simulink model "simulation_ex_4_2014a"  (R2014a)
settings: Solver=ode45  SolverMode=SingleTasking  StartTime=0.0  StopTime=3000  RelTol=1e-3
settings Model: CovMetricSettings=dwe  CovHtmlReporting=off  covSaveCumulativeToWorkspaceVar=off  CovSaveSingleToWorkspaceVar=off  CovExternalEMLEnable=on  CovSFcnEnable=on  Creator=HanO  LastModifiedBy=HanO
settings DataIOCC: LimitDataPoints=off  SaveFormat=StructureWithTime  ReturnWorkspaceOutputs=on
settings DebuggingCC: MergeDetectMultiDrivingBlocksExec=error  SolverPrmCheckMsg=none  FrameProcessingCompatibilityMsg=error  SFUnexpectedBacktrackingDiag=error  SFNoUnconditionalDefaultTransitionDiag=error
settings HardwareCC: ProdBitPerPointer=64  ProdLargestAtomicFloat=Float  ProdIntDivRoundTo=Zero  ProdEndianess=LittleEndian  ProdHWDeviceType=Specified
settings ModelReferenceCC: PropagateSignalLabelsOutOfModel=on
settings SFSimCC: SimUseLocalCustomCode=on
settings RTWCC: RTWUseLocalCustomCode=on
settings GRTTargetCC: TargetLangStandard=C99 (ISO)

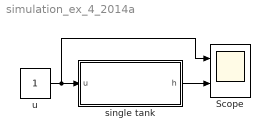
== system simulation_ex_4_2014a ==
  Scope : Scope  NumInputPorts=2
      settings: TimeRange=auto  MaxDataPoints=5000  SaveName=ScopeData  YMin=0.9~-0.19266  YMax=1.1~2.24363  SampleTime=-1
  single tank : Subsystem  mask{AA=50, a=0.5, k=0.1, Cd=0.2, g=9.81, h0=2}
      mask prompts: AA "Tiết diện ngang bồn chứa A ="; a "Tiết diện van xả a ="; k "Hệ số tỉ lệ công suất máy bơm k ="; Cd "Hệ số xả Cd ="; g "Gia tốc trọng trường g ="; h0 "Mực nước ban đầu h0 ="
  u : Constant
  wires:
  u/1 -> Scope/1, single tank/1(u)
  single tank/1(h) -> Scope/2

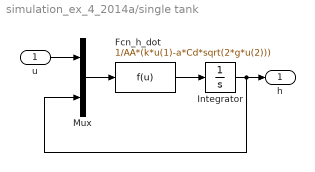
== system simulation_ex_4_2014a/single tank ==
  u : Inport
  Fcn_h_dot : Fcn  Expr=1/AA*(k*u(1)-a*Cd*sqrt(2*g*u(2)))
  Integrator : Integrator  InitialCondition=h0
  Mux : Mux  Inputs=2
  h : Outport
  wires:
  Mux/1 -> Fcn_h_dot/1
  Fcn_h_dot/1 -> Integrator/1
  Integrator/1 -> h/1, Mux/2
  u/1 -> Mux/1
